simulink model "DvrSimKeybd_cs"  (R2016a)
settings: Solver=ode5  SolverMode=SingleTasking  StartTime=0.0  StopTime=10  FixedStep=1/1000  RelTol=1e-3
PreLoadFcn:
  | mbxruntime.callbacks.PreLoadFcn(bdroot);
PostLoadFcn:
  | mbxruntime.callbacks.PostLoadFcn(bdroot);
InitFcn:
  | mbxruntime.callbacks.InitFcn(bdroot);
StartFcn:
  | mbxruntime.callbacks.StartFcn(bdroot);
StopFcn:
  | mbxruntime.callbacks.StopFcn(bdroot);
model workspace (MAT data in the model file):
  mbox_table : struct (value not decoded)
  model_closed = 0
  sim_status = 0
values from neighbouring files (symbols this model uses):
  CCCDuration = 5    [PreScan_Runscript.m]
  V0 = CCCArray(2*CCCCasei-1)    [PreScan_Runscript.m]
  V1 = CCCArray(2*CCCCasei)    [PreScan_Runscript.m]
  VAccuracyIn = 0.8    [PreScan_Runscript.m]
  VDurationIn = 2    [PreScan_Runscript.m]
  VPIDIn = CCCArray(2*CCCCasei-1)    [PreScan_Runscript.m]
  VToleranceIn = 1    [PreScan_Runscript.m]
undefined symbols (not defined in the file or in its folder): ADASID, BMotor1, BMotor2, BrkDelayTime, DControlB, Delay1, Delay2, DiscIntNeverNeededParam, IControlB, JMotor1, JMotor2, PControlB, PreScanCarSimLoadFcn, ratioGearF, ratioGearR, TorqDelayTime, Tstep
undefined symbols (not defined in the file): WheelL0, WheelL1, WheelR0, WheelR1
libraries: simulink x13, simulink_extras x10, MyLib x3, PreScanSimulinkLibrary x3, Solver_SF x2, pil_lib x1
(part 8 of 9)

== system DvrSimKeybd_cs/Roewe_550_S_Sedan_1/CarSim I//O/PreScanLaneMarker/Subsystem/Sensor Data4 ==
  Sensor Data : Inport
  Bus Selector : BusSelector  OutputSignals=ScanAtSensor.LeftLaneIntersection2.WorldCoordinateY,ScanAtDistance1.LeftLaneIntersection2.WorldCoordinateY,ScanAtDistance2.LeftLaneIntersection2.WorldCoordinateY,ScanAtDistance3.LeftLaneIntersection2.WorldCoordinateY
  Bus Selector1 : BusSelector  OutputSignals=ScanAtSensor.LeftLaneIntersection1.WorldCoordinateY,ScanAtDistance1.LeftLaneIntersection1.WorldCoordinateY,ScanAtDistance2.LeftLaneIntersection1.WorldCoordinateY,ScanAtDistance3.LeftLaneIntersection1.WorldCoordinateY
  Bus Selector2 : BusSelector  OutputSignals=ScanAtSensor.RightLaneIntersection1.WorldCoordinateY,ScanAtDistance1.RightLaneIntersection1.WorldCoordinateY,ScanAtDistance2.RightLaneIntersection1.WorldCoordinateY,ScanAtDistance3.RightLaneIntersection1.WorldCoordinateY
  Bus Selector3 : BusSelector  OutputSignals=ScanAtSensor.RightLaneIntersection2.WorldCoordinateX,ScanAtDistance1.RightLaneIntersection2.WorldCoordinateX,ScanAtDistance2.RightLaneIntersection2.WorldCoordinateX,ScanAtDistance3.RightLaneIntersection2.WorldCoordinateX
  Bus Selector5 : BusSelector  OutputSignals=ScanAtSensor.LeftLaneIntersection2.WorldCoordinateX,ScanAtDistance1.LeftLaneIntersection2.WorldCoordinateX,ScanAtDistance2.LeftLaneIntersection2.WorldCoordinateX,ScanAtDistance3.LeftLaneIntersection2.WorldCoordinateX
  Bus Selector6 : BusSelector  OutputSignals=ScanAtSensor.LeftLaneIntersection1.WorldCoordinateX,ScanAtDistance1.LeftLaneIntersection1.WorldCoordinateX,ScanAtDistance2.LeftLaneIntersection1.WorldCoordinateX,ScanAtDistance3.LeftLaneIntersection1.WorldCoordinateX
  Bus Selector7 : BusSelector  OutputSignals=ScanAtSensor.RightLaneIntersection1.WorldCoordinateX,ScanAtDistance1.RightLaneIntersection1.WorldCoordinateX,ScanAtDistance2.RightLaneIntersection1.WorldCoordinateX,ScanAtDistance3.RightLaneIntersection1.WorldCoordinateX
  Bus Selector8 : BusSelector  OutputSignals=ScanAtSensor.RightLaneIntersection2.WorldCoordinateY,ScanAtDistance1.RightLaneIntersection2.WorldCoordinateY,ScanAtDistance2.RightLaneIntersection2.WorldCoordinateY,ScanAtDistance3.RightLaneIntersection2.WorldCoordinateY
  Mux{,1..7} (8 alike) : Mux
  Lane3_X_Part4 : Outport
  Lane1_X_Part4 : Outport  Port=2
  Lane2_X_Part4 : Outport  Port=3
  Lane4_X_Part4 : Outport  Port=4
  Lane3_Y_Part4 : Outport  Port=5
  Lane1_Y_Part4 : Outport  Port=6
  Lane2_Y_Part4 : Outport  Port=7
  Lane4_Y_Part4 : Outport  Port=8
  wires:
  Sensor Data/1 -> Bus Selector8/1, Bus Selector2/1, Bus Selector1/1, Bus Selector/1, Bus Selector3/1, Bus Selector5/1, Bus Selector6/1, Bus Selector7/1
  Bus Selector5/2 -> Mux/2  "<WorldCoordinateX>"
  Bus Selector5/4 -> Mux/4  "<WorldCoordinateX>"
  Bus Selector5/1 -> Mux/1  "<WorldCoordinateX>"
  Bus Selector5/3 -> Mux/3  "<WorldCoordinateX>"
  Bus Selector/3 -> Mux4/3  "<WorldCoordinateY>"
  Bus Selector/4 -> Mux4/4  "<WorldCoordinateY>"
  Bus Selector/1 -> Mux4/1  "<WorldCoordinateY>"
  Bus Selector/2 -> Mux4/2  "<WorldCoordinateY>"
  Mux/1 -> Lane3_X_Part4/1
  Mux4/1 -> Lane3_Y_Part4/1
  Bus Selector6/4 -> Mux5/4  "<WorldCoordinateX>"
  Bus Selector6/3 -> Mux5/3  "<WorldCoordinateX>"
  Bus Selector6/2 -> Mux5/2  "<WorldCoordinateX>"
  Bus Selector6/1 -> Mux5/1  "<WorldCoordinateX>"
  Bus Selector1/3 -> Mux1/3  "<WorldCoordinateY>"
  Bus Selector1/2 -> Mux1/2  "<WorldCoordinateY>"
  Bus Selector1/4 -> Mux1/4  "<WorldCoordinateY>"
  Bus Selector1/1 -> Mux1/1  "<WorldCoordinateY>"
  Mux1/1 -> Lane1_Y_Part4/1
  Mux5/1 -> Lane1_X_Part4/1
  Bus Selector7/2 -> Mux2/2  "<WorldCoordinateX>"
  Bus Selector7/3 -> Mux2/3  "<WorldCoordinateX>"
  Bus Selector7/1 -> Mux2/1  "<WorldCoordinateX>"
  Bus Selector7/4 -> Mux2/4  "<WorldCoordinateX>"
  Bus Selector2/2 -> Mux3/2  "<WorldCoordinateY>"
  Bus Selector2/1 -> Mux3/1  "<WorldCoordinateY>"
  Bus Selector2/3 -> Mux3/3  "<WorldCoordinateY>"
  Bus Selector2/4 -> Mux3/4  "<WorldCoordinateY>"
  Bus Selector3/2 -> Mux6/2  "<WorldCoordinateX>"
  Bus Selector3/1 -> Mux6/1  "<WorldCoordinateX>"
  Bus Selector3/3 -> Mux6/3  "<WorldCoordinateX>"
  Bus Selector3/4 -> Mux6/4  "<WorldCoordinateX>"
  Bus Selector8/1 -> Mux7/1  "<WorldCoordinateY>"
  Bus Selector8/2 -> Mux7/2  "<WorldCoordinateY>"
  Bus Selector8/3 -> Mux7/3  "<WorldCoordinateY>"
  Bus Selector8/4 -> Mux7/4  "<WorldCoordinateY>"
  Mux3/1 -> Lane2_Y_Part4/1
  Mux7/1 -> Lane4_Y_Part4/1
  Mux2/1 -> Lane2_X_Part4/1
  Mux6/1 -> Lane4_X_Part4/1

== system DvrSimKeybd_cs/Roewe_550_S_Sedan_1/CarSim_Vehicle/CarSim2PreScan_BUS/Steering/AvoidDivisionByZero ==
  In1 : Inport
  Compare To Zero : simulink/Logic and Bit Operations/Compare To Zero  relop===  OutDataTypeStr=uint8
  Constant : Constant  Value=eps
  Product : Product  RndMeth=Zero
  Sum : Sum
  Out1 : Outport
  wires:
  In1/1 -> Compare To Zero/1, Sum/1
  Sum/1 -> Out1/1
  Product/1 -> Sum/2
  Constant/1 -> Product/2
  Compare To Zero/1 -> Product/1

== system DvrSimKeybd_cs/Roewe_550_S_Sedan_1/CarSim_Vehicle/CarSim2PreScan_BUS/Wheel/Convert CarSim to PreScan Wheel Position ==
  SprungMass_Pos_Global[x;y;z][m] : Inport
  SprungMass_Angle_Global[x;y;z][deg] : Inport  Port=2
  CarSim_Pos_FL_Wheel[x;y;z][m] : Inport  Port=3
  CarSim_Pos_FR_Wheel[x;y;z][m] : Inport  Port=4
  CarSim_Pos_RL_Wheel[x;y;z][m] : Inport  Port=5
  CarSim_Pos_RR_Wheel[x;y;z][m] : Inport  Port=6
  Bus Creator1 : BusCreator  Inputs=4
  Demux1 : Demux  Outputs=[3 3 3 3]
  Mux1 : Mux
  Transformation_WheelGlobal2WheelLocal : Subsystem
  PreScanWheel_Pos : Outport
  wires:
  SprungMass_Angle_Global[x;y;z][deg]/1 -> Transformation_WheelGlobal2WheelLocal/2(SprungMass_Angle_Global[x;y;z][deg])
  SprungMass_Pos_Global[x;y;z][m]/1 -> Transformation_WheelGlobal2WheelLocal/1(SprungMass_Pos_Global[x;y;z][m])
  CarSim_Pos_RR_Wheel[x;y;z][m]/1 -> Mux1/4
  CarSim_Pos_RL_Wheel[x;y;z][m]/1 -> Mux1/3
  CarSim_Pos_FR_Wheel[x;y;z][m]/1 -> Mux1/2
  CarSim_Pos_FL_Wheel[x;y;z][m]/1 -> Mux1/1
  Mux1/1 -> Transformation_WheelGlobal2WheelLocal/3(Wheels_Pos_Global[x;y;z][m])
  Bus Creator1/1 -> PreScanWheel_Pos/1  "Linear"
  Demux1/4 -> Bus Creator1/4  "Pos_RR_Wheel_CoorSys_V[x;y;z][m]"
  Demux1/3 -> Bus Creator1/3  "Pos_RL_Wheel_CoorSys_V[x;y;z][m]"
  Demux1/2 -> Bus Creator1/2  "Pos_FR_Wheel_CoorSys_V[x;y;z][m]"
  Demux1/1 -> Bus Creator1/1  "Pos_FL_Wheel_CoorSys_V[x;y;z][m]"
  Transformation_WheelGlobal2WheelLocal/1(Pos_[FL;FR;RL;RR]_Wheel_CoorSys_V[x;y;z][m]) -> Demux1/1

== system DvrSimKeybd_cs/Roewe_550_S_Sedan_1/CarSim_Vehicle/CarSim2PreScan_BUS/Wheel/Convert CarSim to PreScan Wheel Rotation ==
  CarSim_Angle_FL_Wheel_CoorSys_V[deg;rev;deg] : Inport
  CarSim_Angle_FR_Wheel_CoorSys_V[deg;rev;deg] : Inport  Port=2
  CarSim_Angle_RL_Wheel_CoorSys_V[deg;rev;deg] : Inport  Port=3
  CarSim_Angle_RR_Wheel_CoorSys_V[deg;rev;deg] : Inport  Port=4
  Angle_Vehicle[x;y;z][deg] : Inport  Port=5
  Bus Creator{,1,3..4} (4 alike) : BusCreator  Inputs=3
  Bus Creator2 : BusCreator  Inputs=4
  Demux{,1..4} (5 alike) : Demux  Outputs=3
  Rev2D{,1..3} (4 alike) : Gain  Gain=360
  Sum{1..4} (4 alike) : Sum  Inputs=+-
  Terminator : Terminator
  Terminator1 : Terminator
  PreScanWheel_Rot : Outport
  wires:
  [VehicleRoll_deg] -> Sum3/2
  Sum3/1 -> Bus Creator4/1  "Angle_Camber_RR_Wheel_CoorSys_V[deg]"
  [VehicleRoll_deg] -> Sum2/2
  Sum1/1 -> Bus Creator1/1  "Angle_Camber_FR_Wheel_CoorSys_V[deg]"
  [VehicleRoll_deg] -> Sum1/2
  [VehicleRoll_deg] -> Sum4/2
  Demux4/3 -> Terminator1/1
  Demux4/2 -> Terminator/1
  Demux4/1 -> [VehicleRoll_deg]
  Angle_Vehicle[x;y;z][deg]/1 -> Demux4/1
  Rev2D3/1 -> Bus Creator4/2  "Angle_Rot_RR_Wheel[deg]"
  Rev2D2/1 -> Bus Creator3/2  "Angle_Rot_RL_Wheel[deg]"
  Rev2D1/1 -> Bus Creator1/2  "Angle_Rot_FR_Wheel[deg]"
  Rev2D/1 -> Bus Creator/2  "Angle_Rot_FL_Wheel[deg]"
  CarSim_Angle_RR_Wheel_CoorSys_V[deg;rev;deg]/1 -> Demux3/1
  CarSim_Angle_RL_Wheel_CoorSys_V[deg;rev;deg]/1 -> Demux2/1
  CarSim_Angle_FR_Wheel_CoorSys_V[deg;rev;deg]/1 -> Demux1/1
  Demux/1 -> Sum4/1  "CarSImAngle_Camber_FL_Wheel_CoorSys_V[deg]"
  Bus Creator2/1 -> PreScanWheel_Rot/1  "Angualr"
  Bus Creator4/1 -> Bus Creator2/4  "Rot_RR_Wheel_CoorSys_V[x;y;z][deg]"
  Bus Creator3/1 -> Bus Creator2/3  "Rot_RL_Wheel_CoorSys_V[x;y;z][deg]"
  Bus Creator1/1 -> Bus Creator2/2  "Rot_FR_Wheel_CoorSys_V[x;y;z][deg]"
  Bus Creator/1 -> Bus Creator2/1  "Rot_FL_Wheel_CoorSys_V[x;y;z][deg]"
  Demux3/3 -> Bus Creator4/3  "Angle_Toe_RR_Wheel_CoorSys_V[deg]"
  Demux1/3 -> Bus Creator1/3  "Angle_Toe_FR_Wheel_CoorSys_V[deg]"
  Demux2/3 -> Bus Creator3/3  "Angle_Toe_RL_Wheel_CoorSys_V[deg]"
  Sum2/1 -> Bus Creator3/1  "Angle_Camber_RL_Wheel_CoorSys_V[deg]"
  Sum4/1 -> Bus Creator/1  "Angle_Camber_FL_Wheel_CoorSys_V[deg]"
  Demux3/2 -> Rev2D3/1  "Angle_Rot_RR_Wheel[rev]"
  Demux3/1 -> Sum3/1  "Angle_Camber_RR_Wheel_CoorSys_V[deg]"
  Demux2/2 -> Rev2D2/1  "Angle_Rot_RL_Wheel[rev]"
  Demux2/1 -> Sum2/1  "Angle_Camber_RL_Wheel_CoorSys_V[deg]"
  Demux1/2 -> Rev2D1/1  "Angle_Rot_FR_Wheel[rev]"
  Demux1/1 -> Sum1/1  "Angle_Camber_FR_Wheel_CoorSys_V[deg]"
  Demux/3 -> Bus Creator/3  "Angle_Toe_FL_Wheel_CoorSys_V[deg]"
  Demux/2 -> Rev2D/1  "Angle_Rot_FL_Wheel[rev]"
  CarSim_Angle_FL_Wheel_CoorSys_V[deg;rev;deg]/1 -> Demux/1

== system DvrSimKeybd_cs/Roewe_550_S_Sedan_1/CarSim_Vehicle/TyreContact To Road Information/Contact To Road Information/AvoidDivisionByZero ==
  In1 : Inport
  Compare To Zero : simulink/Logic and Bit Operations/Compare To Zero  relop===  OutDataTypeStr=uint8
  Constant : Constant  Value=eps
  Product : Product  RndMeth=Zero
  Sum : Sum
  Out1 : Outport
  wires:
  In1/1 -> Compare To Zero/1, Sum/1
  Sum/1 -> Out1/1
  Product/1 -> Sum/2
  Constant/1 -> Product/2
  Compare To Zero/1 -> Product/1

== system DvrSimKeybd_cs/Roewe_550_S_Sedan_1/CarSim_Vehicle/TyreContact To Road Information/Contact To Road Information/Transformation_PreScan2CarSim ==
  UnitVec_z_CP_CoorSys_PreScan[FL;FR;RL;RR][x;y;z] : Inport
  angles_BODYwrtGLOB_[deg] : Inport  Port=2
  Bus Creator : BusCreator  Inputs=4
  D2R : Gain  Gain=pi/180
  Fcn1 : Fcn  Expr=cos(u(1))*sin(u(2))*sin(u(3))-sin(u(1))*cos(u(3))
  Fcn18 : Fcn  Expr=cos(u(1))*cos(u(2))
  Fcn2 : Fcn  Expr=cos(u(1))*sin(u(2))*cos(u(3))+sin(u(1))*sin(u(3))
  Fcn3 : Fcn  Expr=sin(u(1))*cos(u(2))
  Fcn4 : Fcn  Expr=sin(u(1))*sin(u(2))*sin(u(3))+cos(u(1))*cos(u(3))
  Fcn5 : Fcn  Expr=sin(u(1))*sin(u(2))*cos(u(3))-cos(u(1))*sin(u(3))
  Fcn6 : Fcn  Expr=-sin(u(2))
  Fcn7 : Fcn  Expr=cos(u(2))*sin(u(3))
  Fcn8 : Fcn  Expr=cos(u(2))*cos(u(3))
  Mux2 : Mux  Inputs=9
  Selector : Selector  InputPortWidth=9  IndexOptions=Index vector (dialog)  Indices=[1 2 3]  OutputSizes=1
  Selector1 : Selector  InputPortWidth=9  IndexOptions=Index vector (dialog)  Indices=[4 5 6]  OutputSizes=1
  Selector2 : Selector  InputPortWidth=9  IndexOptions=Index vector (dialog)  Indices=[7 8 9]  OutputSizes=1
  Subsystem : Subsystem
  rot_xyz 2 rot_zyx : Selector  InputPortWidth=3  IndexOptions=Index vector (dialog)  Indices=[3 2 1]  OutputSizes=1
  UnitVec_z_CP_CoorSys _CarSim[FL;FR;RL;RR][x;y;z] : Outport
  wires:
  Fcn18/1 -> Mux2/1
  Fcn3/1 -> Mux2/2
  Fcn6/1 -> Mux2/3
  Fcn1/1 -> Mux2/4
  Fcn4/1 -> Mux2/5
  Fcn7/1 -> Mux2/6
  Fcn2/1 -> Mux2/7
  Fcn5/1 -> Mux2/8
  Fcn8/1 -> Mux2/9
  Mux2/1 -> Selector/1, Selector1/1, Selector2/1  "Inverse RotationMatrix"
  rot_xyz 2 rot_zyx/1 -> Fcn18/1, Fcn3/1, Fcn6/1, Fcn1/1, Fcn4/1, Fcn8/1, Fcn5/1, Fcn2/1, Fcn7/1
  D2R/1 -> rot_xyz 2 rot_zyx/1
  Subsystem/4(UnitVec_z_CP_CoorSys_CarSim[RR][x;y;z]) -> Bus Creator/4
  Subsystem/3(UnitVec_z_CP_CoorSys_CarSim[RL][x;y;z]) -> Bus Creator/3
  Subsystem/2(UnitVec_z_CP_CoorSys_CarSim[FR][x;y;z]) -> Bus Creator/2
  Subsystem/1(UnitVec_z_CP_CoorSys_CarSim[FL][x;y;z]) -> Bus Creator/1
  UnitVec_z_CP_CoorSys_PreScan[FL;FR;RL;RR][x;y;z]/1 -> Subsystem/1(UnitVec_z_CP_CoorSys_PreScan[FL;FR;RL;RR][x;y;z])
  angles_BODYwrtGLOB_[deg]/1 -> D2R/1
  Bus Creator/1 -> UnitVec_z_CP_CoorSys _CarSim[FL;FR;RL;RR][x;y;z]/1
  Selector2/1 -> Subsystem/4(ThirdRow)
  Selector1/1 -> Subsystem/3(SecondRow)
  Selector/1 -> Subsystem/2(FirstRow)

== system DvrSimKeybd_cs/Roewe_550_S_Sedan_1/PreScan_RayCast_Contact_Sensor/Vehicle Local to World/state2FullState/Transformation_BODY2GLOBAL1 ==
  POSvector_BODY_[m] : Inport
  angles_BODYwrtGLOB_[rad] : Inport  Port=2
  Dot Product : DotProduct  InputSameDT=on  OutDataTypeStr=Inherit: Inherit via internal rule
  Dot Product1 : DotProduct  InputSameDT=on  OutDataTypeStr=Inherit: Inherit via internal rule
  Dot Product2 : DotProduct  InputSameDT=on  OutDataTypeStr=Inherit: Inherit via internal rule
  Fcn10 : Fcn  Expr=cos(u(1))*sin(u(2))*sin(u(3))-sin(u(1))*cos(u(3))
  Fcn11 : Fcn  Expr=cos(u(1))*sin(u(2))*cos(u(3))+sin(u(1))*sin(u(3))
  Fcn12 : Fcn  Expr=sin(u(1))*cos(u(2))
  Fcn13 : Fcn  Expr=sin(u(1))*sin(u(2))*sin(u(3))+cos(u(1))*cos(u(3))
  Fcn14 : Fcn  Expr=sin(u(1))*sin(u(2))*cos(u(3))-cos(u(1))*sin(u(3))
  Fcn15 : Fcn  Expr=-sin(u(2))
  Fcn16 : Fcn  Expr=cos(u(2))*sin(u(3))
  Fcn17 : Fcn  Expr=cos(u(2))*cos(u(3))
  Fcn9 : Fcn  Expr=cos(u(1))*cos(u(2))
  Mux1 : Mux  Inputs=9
  Mux3 : Mux  Inputs=3
  Selector : Selector  InputPortWidth=9  IndexOptions=Index vector (dialog)  Indices=[1 2 3]  OutputSizes=1
  Selector1 : Selector  InputPortWidth=9  IndexOptions=Index vector (dialog)  Indices=[4 5 6]  OutputSizes=1
  Selector2 : Selector  InputPortWidth=9  IndexOptions=Index vector (dialog)  Indices=[7 8 9]  OutputSizes=1
  rot_xyz 2 rot_zyx : Selector  InputPortWidth=3  IndexOptions=Index vector (dialog)  Indices=[3 2 1]  OutputSizes=1
  POSvector_GLOBAL_[m] : Outport
  wires:
  angles_BODYwrtGLOB_[rad]/1 -> rot_xyz 2 rot_zyx/1
  Mux3/1 -> POSvector_GLOBAL_[m]/1
  rot_xyz 2 rot_zyx/1 -> Fcn17/1, Fcn16/1, Fcn15/1, Fcn14/1, Fcn13/1, Fcn12/1, Fcn11/1, Fcn10/1, Fcn9/1
  Dot Product1/1 -> Mux3/2
  Dot Product2/1 -> Mux3/3
  Selector2/1 -> Dot Product2/2
  Selector1/1 -> Dot Product1/2
  Dot Product/1 -> Mux3/1
  POSvector_BODY_[m]/1 -> Dot Product/1, Dot Product1/1, Dot Product2/1
  Selector/1 -> Dot Product/2
  Mux1/1 -> Selector2/1, Selector1/1, Selector/1  "RotationMatrix"
  Fcn17/1 -> Mux1/9
  Fcn16/1 -> Mux1/8
  Fcn15/1 -> Mux1/7
  Fcn14/1 -> Mux1/6
  Fcn13/1 -> Mux1/5
  Fcn12/1 -> Mux1/4
  Fcn11/1 -> Mux1/3
  Fcn10/1 -> Mux1/2
  Fcn9/1 -> Mux1/1

== system DvrSimKeybd_cs/Roewe_550_S_Sedan_1/PreScan_RayCast_Contact_Sensor/Vehicle Local to World/state2FullState/limit roll ==
  RPY : Inport
  Demux : Demux  Outputs=3
  Mux1 : Mux  Inputs=3
  Substitute 90 & 270 deg (and its plurals) : Subsystem
  RPYcor : Outport
  wires:
  Demux/1 -> Substitute 90 & 270 deg (and its plurals)/1(Angle [rad])
  Demux/2 -> Mux1/2
  Demux/3 -> Mux1/3
  RPY/1 -> Demux/1
  Mux1/1 -> RPYcor/1
  Substitute 90 & 270 deg (and its plurals)/1(Subst Angle [rad]) -> Mux1/1

== system DvrSimKeybd_cs/Roewe_550_S_Sedan_1/PreScan_RayCast_Contact_Sensor/Wheels Local to World/conv_RotWheelFL/RotMat2AxisAngle ==
  RotMat_Visu : Inport
  Data Type Conversion : DataTypeConversion
  Divide : Product  Inputs=*/
  Gain : Gain  Gain=2
  Mux : Mux  Inputs=3
  Mux1 : Mux  Inputs=2
  Saturation1 : Saturate  UpperLimit=3-0.001  LowerLimit=-1+0.001
  Trigonometric Function : Trigonometry
  U1 : Fcn  Expr=u[6]-u[8]
  U2 : Fcn  Expr=u[7]-u[3]
  U3 : Fcn  Expr=u[2]-u[4]
  U_Phi : Fcn  Expr=u[1]+u[5]+u[9]
  U_Phi1 : Fcn  Expr=acos((u(1)-1)/2)
  U_Phi2 : Fcn  Expr=acos((u(1)-1)/2)
  Angles_Visu : Outport
  wires:
  Data Type Conversion/1 -> Mux1/2
  RotMat_Visu/1 -> U1/1, U2/1, U3/1, U_Phi/1
  Trigonometric Function/1 -> Gain/1
  U1/1 -> Mux/1
  U2/1 -> Mux/2
  U3/1 -> Mux/3
  Mux/1 -> Divide/1
  Gain/1 -> Divide/2
  Mux1/1 -> Angles_Visu/1
  Divide/1 -> Mux1/1
  U_Phi/1 -> U_Phi1/1, Saturation1/1
  U_Phi1/1 -> Data Type Conversion/1
  Saturation1/1 -> U_Phi2/1
  U_Phi2/1 -> Trigonometric Function/1

== system DvrSimKeybd_cs/Roewe_550_S_Sedan_1/PreScan_RayCast_Contact_Sensor/Wheels Local to World/conv_RotWheelFR/RotMat2AxisAngle ==
  RotMat_Visu : Inport
  Data Type Conversion : DataTypeConversion
  Divide : Product  Inputs=*/
  Gain : Gain  Gain=2
  Mux : Mux  Inputs=3
  Mux1 : Mux  Inputs=2
  Saturation1 : Saturate  UpperLimit=3-0.001  LowerLimit=-1+0.001
  Trigonometric Function : Trigonometry
  U1 : Fcn  Expr=u[6]-u[8]
  U2 : Fcn  Expr=u[7]-u[3]
  U3 : Fcn  Expr=u[2]-u[4]
  U_Phi : Fcn  Expr=u[1]+u[5]+u[9]
  U_Phi1 : Fcn  Expr=acos((u(1)-1)/2)
  U_Phi2 : Fcn  Expr=acos((u(1)-1)/2)
  Angles_Visu : Outport
  wires:
  U_Phi2/1 -> Trigonometric Function/1
  Saturation1/1 -> U_Phi2/1
  U_Phi1/1 -> Data Type Conversion/1
  U_Phi/1 -> Saturation1/1, U_Phi1/1
  Divide/1 -> Mux1/1
  Mux1/1 -> Angles_Visu/1
  Gain/1 -> Divide/2
  Mux/1 -> Divide/1
  U3/1 -> Mux/3
  U2/1 -> Mux/2
  U1/1 -> Mux/1
  Trigonometric Function/1 -> Gain/1
  RotMat_Visu/1 -> U_Phi/1, U3/1, U2/1, U1/1
  Data Type Conversion/1 -> Mux1/2

== system DvrSimKeybd_cs/Roewe_550_S_Sedan_1/PreScan_RayCast_Contact_Sensor/Wheels Local to World/conv_RotWheelRL/RotMat2AxisAngle ==
  RotMat_Visu : Inport
  Data Type Conversion : DataTypeConversion
  Divide : Product  Inputs=*/
  Gain : Gain  Gain=2
  Mux : Mux  Inputs=3
  Mux1 : Mux  Inputs=2
  Saturation1 : Saturate  UpperLimit=3-0.001  LowerLimit=-1+0.001
  Trigonometric Function : Trigonometry
  U1 : Fcn  Expr=u[6]-u[8]
  U2 : Fcn  Expr=u[7]-u[3]
  U3 : Fcn  Expr=u[2]-u[4]
  U_Phi : Fcn  Expr=u[1]+u[5]+u[9]
  U_Phi1 : Fcn  Expr=acos((u(1)-1)/2)
  U_Phi2 : Fcn  Expr=acos((u(1)-1)/2)
  Angles_Visu : Outport
  wires:
  U_Phi2/1 -> Trigonometric Function/1
  Saturation1/1 -> U_Phi2/1
  U_Phi1/1 -> Data Type Conversion/1
  U_Phi/1 -> Saturation1/1, U_Phi1/1
  Divide/1 -> Mux1/1
  Mux1/1 -> Angles_Visu/1
  Gain/1 -> Divide/2
  Mux/1 -> Divide/1
  U3/1 -> Mux/3
  U2/1 -> Mux/2
  U1/1 -> Mux/1
  Trigonometric Function/1 -> Gain/1
  RotMat_Visu/1 -> U_Phi/1, U3/1, U2/1, U1/1
  Data Type Conversion/1 -> Mux1/2

== system DvrSimKeybd_cs/Roewe_550_S_Sedan_1/PreScan_RayCast_Contact_Sensor/Wheels Local to World/conv_RotWheelRR/RotMat2AxisAngle ==
  RotMat_Visu : Inport
  Data Type Conversion : DataTypeConversion
  Divide : Product  Inputs=*/
  Gain : Gain  Gain=2
  Mux : Mux  Inputs=3
  Mux1 : Mux  Inputs=2
  Saturation1 : Saturate  UpperLimit=3-0.001  LowerLimit=-1+0.001
  Trigonometric Function : Trigonometry
  U1 : Fcn  Expr=u[6]-u[8]
  U2 : Fcn  Expr=u[7]-u[3]
  U3 : Fcn  Expr=u[2]-u[4]
  U_Phi : Fcn  Expr=u[1]+u[5]+u[9]
  U_Phi1 : Fcn  Expr=acos((u(1)-1)/2)
  U_Phi2 : Fcn  Expr=acos((u(1)-1)/2)
  Angles_Visu : Outport
  wires:
  U_Phi2/1 -> Trigonometric Function/1
  Saturation1/1 -> U_Phi2/1
  U_Phi1/1 -> Data Type Conversion/1
  U_Phi/1 -> Saturation1/1, U_Phi1/1
  Divide/1 -> Mux1/1
  Mux1/1 -> Angles_Visu/1
  Gain/1 -> Divide/2
  Mux/1 -> Divide/1
  U3/1 -> Mux/3
  U2/1 -> Mux/2
  U1/1 -> Mux/1
  Trigonometric Function/1 -> Gain/1
  RotMat_Visu/1 -> U_Phi/1, U3/1, U2/1, U1/1
  Data Type Conversion/1 -> Mux1/2

== system DvrSimKeybd_cs/Roewe_550_S_Sedan_1/PreScan_RayCast_Contact_Sensor/Wheels Local to World/conv_TransWheelFL/pos_ini_Visu ==
  Constant : Constant  Value=x_ini_VRML
  Constant1 : Constant  Value=y_ini_VRML
  Constant2 : Constant  Value=z_ini_VRML
  Mux1 : Mux  Inputs=3
  pos_ini_Visu : Outport
  wires:
  Constant/1 -> Mux1/1
  Mux1/1 -> pos_ini_Visu/1
  Constant1/1 -> Mux1/2
  Constant2/1 -> Mux1/3

== system DvrSimKeybd_cs/Roewe_550_S_Sedan_1/PreScan_RayCast_Contact_Sensor/Wheels Local to World/conv_TransWheelFL/transISO2Visu ==
  transISO : Inport
  Demux : Demux  Outputs=3
  trans_x_Visu : Outport
  trans_y_Visu : Outport  Port=2
  trans_z_Visu : Outport  Port=3
  wires:
  Demux/2 -> trans_y_Visu/1  "rot_y"
  Demux/1 -> trans_x_Visu/1
  transISO/1 -> Demux/1
  Demux/3 -> trans_z_Visu/1

== system DvrSimKeybd_cs/Roewe_550_S_Sedan_1/PreScan_RayCast_Contact_Sensor/Wheels Local to World/conv_TransWheelFR/pos_ini_Visu ==
  Constant : Constant  Value=x_ini_VRML
  Constant1 : Constant  Value=y_ini_VRML
  Constant2 : Constant  Value=z_ini_VRML
  Mux1 : Mux  Inputs=3
  pos_ini_Visu : Outport
  wires:
  Constant2/1 -> Mux1/3
  Constant1/1 -> Mux1/2
  Mux1/1 -> pos_ini_Visu/1
  Constant/1 -> Mux1/1

== system DvrSimKeybd_cs/Roewe_550_S_Sedan_1/PreScan_RayCast_Contact_Sensor/Wheels Local to World/conv_TransWheelFR/transISO2Visu ==
  transISO : Inport
  Demux : Demux  Outputs=3
  trans_x_Visu : Outport
  trans_y_Visu : Outport  Port=2
  trans_z_Visu : Outport  Port=3
  wires:
  Demux/2 -> trans_y_Visu/1  "rot_y"
  Demux/1 -> trans_x_Visu/1
  transISO/1 -> Demux/1
  Demux/3 -> trans_z_Visu/1

== system DvrSimKeybd_cs/Roewe_550_S_Sedan_1/PreScan_RayCast_Contact_Sensor/Wheels Local to World/conv_TransWheelRL/pos_ini_Visu ==
  Constant : Constant  Value=x_ini_VRML
  Constant1 : Constant  Value=y_ini_VRML
  Constant2 : Constant  Value=z_ini_VRML
  Mux1 : Mux  Inputs=3
  pos_ini_Visu : Outport
  wires:
  Constant2/1 -> Mux1/3
  Constant1/1 -> Mux1/2
  Mux1/1 -> pos_ini_Visu/1
  Constant/1 -> Mux1/1

== system DvrSimKeybd_cs/Roewe_550_S_Sedan_1/PreScan_RayCast_Contact_Sensor/Wheels Local to World/conv_TransWheelRL/transISO2Visu ==
  transISO : Inport
  Demux : Demux  Outputs=3
  trans_x_Visu : Outport
  trans_y_Visu : Outport  Port=2
  trans_z_Visu : Outport  Port=3
  wires:
  Demux/2 -> trans_y_Visu/1  "rot_y"
  Demux/1 -> trans_x_Visu/1
  transISO/1 -> Demux/1
  Demux/3 -> trans_z_Visu/1

== system DvrSimKeybd_cs/Roewe_550_S_Sedan_1/PreScan_RayCast_Contact_Sensor/Wheels Local to World/conv_TransWheelRR/pos_ini_Visu ==
  Constant : Constant  Value=x_ini_VRML
  Constant1 : Constant  Value=y_ini_VRML
  Constant2 : Constant  Value=z_ini_VRML
  Mux1 : Mux  Inputs=3
  pos_ini_Visu : Outport
  wires:
  Constant2/1 -> Mux1/3
  Constant1/1 -> Mux1/2
  Mux1/1 -> pos_ini_Visu/1
  Constant/1 -> Mux1/1

== system DvrSimKeybd_cs/Roewe_550_S_Sedan_1/PreScan_RayCast_Contact_Sensor/Wheels Local to World/conv_TransWheelRR/transISO2Visu ==
  transISO : Inport
  Demux : Demux  Outputs=3
  trans_x_Visu : Outport
  trans_y_Visu : Outport  Port=2
  trans_z_Visu : Outport  Port=3
  wires:
  Demux/2 -> trans_y_Visu/1  "rot_y"
  Demux/1 -> trans_x_Visu/1
  transISO/1 -> Demux/1
  Demux/3 -> trans_z_Visu/1

== system DvrSimKeybd_cs/Roewe_550_S_Sedan_1/PreScan_RayCast_Contact_Sensor1/Vehicle Local to World/state2FullState/Transformation_BODY2GLOBAL1 ==
  POSvector_BODY_[m] : Inport
  angles_BODYwrtGLOB_[rad] : Inport  Port=2
  Dot Product : DotProduct  InputSameDT=on  OutDataTypeStr=Inherit: Inherit via internal rule
  Dot Product1 : DotProduct  InputSameDT=on  OutDataTypeStr=Inherit: Inherit via internal rule
  Dot Product2 : DotProduct  InputSameDT=on  OutDataTypeStr=Inherit: Inherit via internal rule
  Fcn10 : Fcn  Expr=cos(u(1))*sin(u(2))*sin(u(3))-sin(u(1))*cos(u(3))
  Fcn11 : Fcn  Expr=cos(u(1))*sin(u(2))*cos(u(3))+sin(u(1))*sin(u(3))
  Fcn12 : Fcn  Expr=sin(u(1))*cos(u(2))
  Fcn13 : Fcn  Expr=sin(u(1))*sin(u(2))*sin(u(3))+cos(u(1))*cos(u(3))
  Fcn14 : Fcn  Expr=sin(u(1))*sin(u(2))*cos(u(3))-cos(u(1))*sin(u(3))
  Fcn15 : Fcn  Expr=-sin(u(2))
  Fcn16 : Fcn  Expr=cos(u(2))*sin(u(3))
  Fcn17 : Fcn  Expr=cos(u(2))*cos(u(3))
  Fcn9 : Fcn  Expr=cos(u(1))*cos(u(2))
  Mux1 : Mux  Inputs=9
  Mux3 : Mux  Inputs=3
  Selector : Selector  InputPortWidth=9  IndexOptions=Index vector (dialog)  Indices=[1 2 3]  OutputSizes=1
  Selector1 : Selector  InputPortWidth=9  IndexOptions=Index vector (dialog)  Indices=[4 5 6]  OutputSizes=1
  Selector2 : Selector  InputPortWidth=9  IndexOptions=Index vector (dialog)  Indices=[7 8 9]  OutputSizes=1
  rot_xyz 2 rot_zyx : Selector  InputPortWidth=3  IndexOptions=Index vector (dialog)  Indices=[3 2 1]  OutputSizes=1
  POSvector_GLOBAL_[m] : Outport
  wires:
  angles_BODYwrtGLOB_[rad]/1 -> rot_xyz 2 rot_zyx/1
  Mux3/1 -> POSvector_GLOBAL_[m]/1
  rot_xyz 2 rot_zyx/1 -> Fcn17/1, Fcn16/1, Fcn15/1, Fcn14/1, Fcn13/1, Fcn12/1, Fcn11/1, Fcn10/1, Fcn9/1
  Dot Product1/1 -> Mux3/2
  Dot Product2/1 -> Mux3/3
  Selector2/1 -> Dot Product2/2
  Selector1/1 -> Dot Product1/2
  Dot Product/1 -> Mux3/1
  POSvector_BODY_[m]/1 -> Dot Product/1, Dot Product1/1, Dot Product2/1
  Selector/1 -> Dot Product/2
  Mux1/1 -> Selector2/1, Selector1/1, Selector/1  "RotationMatrix"
  Fcn17/1 -> Mux1/9
  Fcn16/1 -> Mux1/8
  Fcn15/1 -> Mux1/7
  Fcn14/1 -> Mux1/6
  Fcn13/1 -> Mux1/5
  Fcn12/1 -> Mux1/4
  Fcn11/1 -> Mux1/3
  Fcn10/1 -> Mux1/2
  Fcn9/1 -> Mux1/1

== system DvrSimKeybd_cs/Roewe_550_S_Sedan_1/PreScan_RayCast_Contact_Sensor1/Vehicle Local to World/state2FullState/limit roll ==
  RPY : Inport
  Demux : Demux  Outputs=3
  Mux1 : Mux  Inputs=3
  Substitute 90 & 270 deg (and its plurals) : Subsystem
  RPYcor : Outport
  wires:
  Demux/1 -> Substitute 90 & 270 deg (and its plurals)/1(Angle [rad])
  Demux/2 -> Mux1/2
  Demux/3 -> Mux1/3
  RPY/1 -> Demux/1
  Mux1/1 -> RPYcor/1
  Substitute 90 & 270 deg (and its plurals)/1(Subst Angle [rad]) -> Mux1/1

== system DvrSimKeybd_cs/Roewe_550_S_Sedan_1/PreScan_RayCast_Contact_Sensor1/Wheels Local to World/conv_RotWheelFL/RotMat2AxisAngle ==
  RotMat_Visu : Inport
  Data Type Conversion : DataTypeConversion
  Divide : Product  Inputs=*/
  Gain : Gain  Gain=2
  Mux : Mux  Inputs=3
  Mux1 : Mux  Inputs=2
  Saturation1 : Saturate  UpperLimit=3-0.001  LowerLimit=-1+0.001
  Trigonometric Function : Trigonometry
  U1 : Fcn  Expr=u[6]-u[8]
  U2 : Fcn  Expr=u[7]-u[3]
  U3 : Fcn  Expr=u[2]-u[4]
  U_Phi : Fcn  Expr=u[1]+u[5]+u[9]
  U_Phi1 : Fcn  Expr=acos((u(1)-1)/2)
  U_Phi2 : Fcn  Expr=acos((u(1)-1)/2)
  Angles_Visu : Outport
  wires:
  Data Type Conversion/1 -> Mux1/2
  RotMat_Visu/1 -> U1/1, U2/1, U3/1, U_Phi/1
  Trigonometric Function/1 -> Gain/1
  U1/1 -> Mux/1
  U2/1 -> Mux/2
  U3/1 -> Mux/3
  Mux/1 -> Divide/1
  Gain/1 -> Divide/2
  Mux1/1 -> Angles_Visu/1
  Divide/1 -> Mux1/1
  U_Phi/1 -> U_Phi1/1, Saturation1/1
  U_Phi1/1 -> Data Type Conversion/1
  Saturation1/1 -> U_Phi2/1
  U_Phi2/1 -> Trigonometric Function/1

== system DvrSimKeybd_cs/Roewe_550_S_Sedan_1/PreScan_RayCast_Contact_Sensor1/Wheels Local to World/conv_RotWheelFR/RotMat2AxisAngle ==
  RotMat_Visu : Inport
  Data Type Conversion : DataTypeConversion
  Divide : Product  Inputs=*/
  Gain : Gain  Gain=2
  Mux : Mux  Inputs=3
  Mux1 : Mux  Inputs=2
  Saturation1 : Saturate  UpperLimit=3-0.001  LowerLimit=-1+0.001
  Trigonometric Function : Trigonometry
  U1 : Fcn  Expr=u[6]-u[8]
  U2 : Fcn  Expr=u[7]-u[3]
  U3 : Fcn  Expr=u[2]-u[4]
  U_Phi : Fcn  Expr=u[1]+u[5]+u[9]
  U_Phi1 : Fcn  Expr=acos((u(1)-1)/2)
  U_Phi2 : Fcn  Expr=acos((u(1)-1)/2)
  Angles_Visu : Outport
  wires:
  U_Phi2/1 -> Trigonometric Function/1
  Saturation1/1 -> U_Phi2/1
  U_Phi1/1 -> Data Type Conversion/1
  U_Phi/1 -> Saturation1/1, U_Phi1/1
  Divide/1 -> Mux1/1
  Mux1/1 -> Angles_Visu/1
  Gain/1 -> Divide/2
  Mux/1 -> Divide/1
  U3/1 -> Mux/3
  U2/1 -> Mux/2
  U1/1 -> Mux/1
  Trigonometric Function/1 -> Gain/1
  RotMat_Visu/1 -> U_Phi/1, U3/1, U2/1, U1/1
  Data Type Conversion/1 -> Mux1/2

== system DvrSimKeybd_cs/Roewe_550_S_Sedan_1/PreScan_RayCast_Contact_Sensor1/Wheels Local to World/conv_RotWheelRL/RotMat2AxisAngle ==
  RotMat_Visu : Inport
  Data Type Conversion : DataTypeConversion
  Divide : Product  Inputs=*/
  Gain : Gain  Gain=2
  Mux : Mux  Inputs=3
  Mux1 : Mux  Inputs=2
  Saturation1 : Saturate  UpperLimit=3-0.001  LowerLimit=-1+0.001
  Trigonometric Function : Trigonometry
  U1 : Fcn  Expr=u[6]-u[8]
  U2 : Fcn  Expr=u[7]-u[3]
  U3 : Fcn  Expr=u[2]-u[4]
  U_Phi : Fcn  Expr=u[1]+u[5]+u[9]
  U_Phi1 : Fcn  Expr=acos((u(1)-1)/2)
  U_Phi2 : Fcn  Expr=acos((u(1)-1)/2)
  Angles_Visu : Outport
  wires:
  U_Phi2/1 -> Trigonometric Function/1
  Saturation1/1 -> U_Phi2/1
  U_Phi1/1 -> Data Type Conversion/1
  U_Phi/1 -> Saturation1/1, U_Phi1/1
  Divide/1 -> Mux1/1
  Mux1/1 -> Angles_Visu/1
  Gain/1 -> Divide/2
  Mux/1 -> Divide/1
  U3/1 -> Mux/3
  U2/1 -> Mux/2
  U1/1 -> Mux/1
  Trigonometric Function/1 -> Gain/1
  RotMat_Visu/1 -> U_Phi/1, U3/1, U2/1, U1/1
  Data Type Conversion/1 -> Mux1/2

== system DvrSimKeybd_cs/Roewe_550_S_Sedan_1/PreScan_RayCast_Contact_Sensor1/Wheels Local to World/conv_RotWheelRR/RotMat2AxisAngle ==
  RotMat_Visu : Inport
  Data Type Conversion : DataTypeConversion
  Divide : Product  Inputs=*/
  Gain : Gain  Gain=2
  Mux : Mux  Inputs=3
  Mux1 : Mux  Inputs=2
  Saturation1 : Saturate  UpperLimit=3-0.001  LowerLimit=-1+0.001
  Trigonometric Function : Trigonometry
  U1 : Fcn  Expr=u[6]-u[8]
  U2 : Fcn  Expr=u[7]-u[3]
  U3 : Fcn  Expr=u[2]-u[4]
  U_Phi : Fcn  Expr=u[1]+u[5]+u[9]
  U_Phi1 : Fcn  Expr=acos((u(1)-1)/2)
  U_Phi2 : Fcn  Expr=acos((u(1)-1)/2)
  Angles_Visu : Outport
  wires:
  U_Phi2/1 -> Trigonometric Function/1
  Saturation1/1 -> U_Phi2/1
  U_Phi1/1 -> Data Type Conversion/1
  U_Phi/1 -> Saturation1/1, U_Phi1/1
  Divide/1 -> Mux1/1
  Mux1/1 -> Angles_Visu/1
  Gain/1 -> Divide/2
  Mux/1 -> Divide/1
  U3/1 -> Mux/3
  U2/1 -> Mux/2
  U1/1 -> Mux/1
  Trigonometric Function/1 -> Gain/1
  RotMat_Visu/1 -> U_Phi/1, U3/1, U2/1, U1/1
  Data Type Conversion/1 -> Mux1/2

== system DvrSimKeybd_cs/Roewe_550_S_Sedan_1/PreScan_RayCast_Contact_Sensor1/Wheels Local to World/conv_TransWheelFL/pos_ini_Visu ==
  Constant : Constant  Value=x_ini_VRML
  Constant1 : Constant  Value=y_ini_VRML
  Constant2 : Constant  Value=z_ini_VRML
  Mux1 : Mux  Inputs=3
  pos_ini_Visu : Outport
  wires:
  Constant/1 -> Mux1/1
  Mux1/1 -> pos_ini_Visu/1
  Constant1/1 -> Mux1/2
  Constant2/1 -> Mux1/3

== system DvrSimKeybd_cs/Roewe_550_S_Sedan_1/PreScan_RayCast_Contact_Sensor1/Wheels Local to World/conv_TransWheelFL/transISO2Visu ==
  transISO : Inport
  Demux : Demux  Outputs=3
  trans_x_Visu : Outport
  trans_y_Visu : Outport  Port=2
  trans_z_Visu : Outport  Port=3
  wires:
  Demux/2 -> trans_y_Visu/1  "rot_y"
  Demux/1 -> trans_x_Visu/1
  transISO/1 -> Demux/1
  Demux/3 -> trans_z_Visu/1

== system DvrSimKeybd_cs/Roewe_550_S_Sedan_1/PreScan_RayCast_Contact_Sensor1/Wheels Local to World/conv_TransWheelFR/pos_ini_Visu ==
  Constant : Constant  Value=x_ini_VRML
  Constant1 : Constant  Value=y_ini_VRML
  Constant2 : Constant  Value=z_ini_VRML
  Mux1 : Mux  Inputs=3
  pos_ini_Visu : Outport
  wires:
  Constant2/1 -> Mux1/3
  Constant1/1 -> Mux1/2
  Mux1/1 -> pos_ini_Visu/1
  Constant/1 -> Mux1/1

== system DvrSimKeybd_cs/Roewe_550_S_Sedan_1/PreScan_RayCast_Contact_Sensor1/Wheels Local to World/conv_TransWheelFR/transISO2Visu ==
  transISO : Inport
  Demux : Demux  Outputs=3
  trans_x_Visu : Outport
  trans_y_Visu : Outport  Port=2
  trans_z_Visu : Outport  Port=3
  wires:
  Demux/2 -> trans_y_Visu/1  "rot_y"
  Demux/1 -> trans_x_Visu/1
  transISO/1 -> Demux/1
  Demux/3 -> trans_z_Visu/1

== system DvrSimKeybd_cs/Roewe_550_S_Sedan_1/PreScan_RayCast_Contact_Sensor1/Wheels Local to World/conv_TransWheelRL/pos_ini_Visu ==
  Constant : Constant  Value=x_ini_VRML
  Constant1 : Constant  Value=y_ini_VRML
  Constant2 : Constant  Value=z_ini_VRML
  Mux1 : Mux  Inputs=3
  pos_ini_Visu : Outport
  wires:
  Constant2/1 -> Mux1/3
  Constant1/1 -> Mux1/2
  Mux1/1 -> pos_ini_Visu/1
  Constant/1 -> Mux1/1

== system DvrSimKeybd_cs/Roewe_550_S_Sedan_1/PreScan_RayCast_Contact_Sensor1/Wheels Local to World/conv_TransWheelRL/transISO2Visu ==
  transISO : Inport
  Demux : Demux  Outputs=3
  trans_x_Visu : Outport
  trans_y_Visu : Outport  Port=2
  trans_z_Visu : Outport  Port=3
  wires:
  Demux/2 -> trans_y_Visu/1  "rot_y"
  Demux/1 -> trans_x_Visu/1
  transISO/1 -> Demux/1
  Demux/3 -> trans_z_Visu/1

== system DvrSimKeybd_cs/Roewe_550_S_Sedan_1/PreScan_RayCast_Contact_Sensor1/Wheels Local to World/conv_TransWheelRR/pos_ini_Visu ==
  Constant : Constant  Value=x_ini_VRML
  Constant1 : Constant  Value=y_ini_VRML
  Constant2 : Constant  Value=z_ini_VRML
  Mux1 : Mux  Inputs=3
  pos_ini_Visu : Outport
  wires:
  Constant2/1 -> Mux1/3
  Constant1/1 -> Mux1/2
  Mux1/1 -> pos_ini_Visu/1
  Constant/1 -> Mux1/1

== system DvrSimKeybd_cs/Roewe_550_S_Sedan_1/PreScan_RayCast_Contact_Sensor1/Wheels Local to World/conv_TransWheelRR/transISO2Visu ==
  transISO : Inport
  Demux : Demux  Outputs=3
  trans_x_Visu : Outport
  trans_y_Visu : Outport  Port=2
  trans_z_Visu : Outport  Port=3
  wires:
  Demux/2 -> trans_y_Visu/1  "rot_y"
  Demux/1 -> trans_x_Visu/1
  transISO/1 -> Demux/1
  Demux/3 -> trans_z_Visu/1

== system DvrSimKeybd_cs/Roewe_550_S_Sedan_1/Subsystem/TyreContact To Road Information/Contact To Road Information/AvoidDivisionByZero ==
  In1 : Inport
  Compare To Zero : simulink/Logic and Bit Operations/Compare To Zero  relop===  OutDataTypeStr=uint8
  Constant : Constant  Value=eps
  Product : Product  RndMeth=Zero
  Sum : Sum
  Out1 : Outport
  wires:
  In1/1 -> Compare To Zero/1, Sum/1
  Sum/1 -> Out1/1
  Product/1 -> Sum/2
  Constant/1 -> Product/2
  Compare To Zero/1 -> Product/1

== system DvrSimKeybd_cs/Roewe_550_S_Sedan_1/Subsystem/TyreContact To Road Information/Contact To Road Information/Transformation_PreScan2CarSim ==
  UnitVec_z_CP_CoorSys_PreScan[FL;FR;RL;RR][x;y;z] : Inport
  angles_BODYwrtGLOB_[deg] : Inport  Port=2
  Bus Creator : BusCreator  Inputs=4
  D2R : Gain  Gain=pi/180
  Fcn1 : Fcn  Expr=cos(u(1))*sin(u(2))*sin(u(3))-sin(u(1))*cos(u(3))
  Fcn18 : Fcn  Expr=cos(u(1))*cos(u(2))
  Fcn2 : Fcn  Expr=cos(u(1))*sin(u(2))*cos(u(3))+sin(u(1))*sin(u(3))
  Fcn3 : Fcn  Expr=sin(u(1))*cos(u(2))
  Fcn4 : Fcn  Expr=sin(u(1))*sin(u(2))*sin(u(3))+cos(u(1))*cos(u(3))
  Fcn5 : Fcn  Expr=sin(u(1))*sin(u(2))*cos(u(3))-cos(u(1))*sin(u(3))
  Fcn6 : Fcn  Expr=-sin(u(2))
  Fcn7 : Fcn  Expr=cos(u(2))*sin(u(3))
  Fcn8 : Fcn  Expr=cos(u(2))*cos(u(3))
  Mux2 : Mux  Inputs=9
  Selector : Selector  InputPortWidth=9  IndexOptions=Index vector (dialog)  Indices=[1 2 3]  OutputSizes=1
  Selector1 : Selector  InputPortWidth=9  IndexOptions=Index vector (dialog)  Indices=[4 5 6]  OutputSizes=1
  Selector2 : Selector  InputPortWidth=9  IndexOptions=Index vector (dialog)  Indices=[7 8 9]  OutputSizes=1
  Subsystem : Subsystem
  rot_xyz 2 rot_zyx : Selector  InputPortWidth=3  IndexOptions=Index vector (dialog)  Indices=[3 2 1]  OutputSizes=1
  UnitVec_z_CP_CoorSys _CarSim[FL;FR;RL;RR][x;y;z] : Outport
  wires:
  Fcn18/1 -> Mux2/1
  Fcn3/1 -> Mux2/2
  Fcn6/1 -> Mux2/3
  Fcn1/1 -> Mux2/4
  Fcn4/1 -> Mux2/5
  Fcn7/1 -> Mux2/6
  Fcn2/1 -> Mux2/7
  Fcn5/1 -> Mux2/8
  Fcn8/1 -> Mux2/9
  Mux2/1 -> Selector/1, Selector1/1, Selector2/1  "Inverse RotationMatrix"
  rot_xyz 2 rot_zyx/1 -> Fcn18/1, Fcn3/1, Fcn6/1, Fcn1/1, Fcn4/1, Fcn8/1, Fcn5/1, Fcn2/1, Fcn7/1
  D2R/1 -> rot_xyz 2 rot_zyx/1
  Subsystem/4(UnitVec_z_CP_CoorSys_CarSim[RR][x;y;z]) -> Bus Creator/4
  Subsystem/3(UnitVec_z_CP_CoorSys_CarSim[RL][x;y;z]) -> Bus Creator/3
  Subsystem/2(UnitVec_z_CP_CoorSys_CarSim[FR][x;y;z]) -> Bus Creator/2
  Subsystem/1(UnitVec_z_CP_CoorSys_CarSim[FL][x;y;z]) -> Bus Creator/1
  UnitVec_z_CP_CoorSys_PreScan[FL;FR;RL;RR][x;y;z]/1 -> Subsystem/1(UnitVec_z_CP_CoorSys_PreScan[FL;FR;RL;RR][x;y;z])
  angles_BODYwrtGLOB_[deg]/1 -> D2R/1
  Bus Creator/1 -> UnitVec_z_CP_CoorSys _CarSim[FL;FR;RL;RR][x;y;z]/1
  Selector2/1 -> Subsystem/4(ThirdRow)
  Selector1/1 -> Subsystem/3(SecondRow)
  Selector/1 -> Subsystem/2(FirstRow)

== system DvrSimKeybd_cs/Roewe_550_S_Sedan_1/Subsystem1/CarSim2PreScan_BUS/Steering/AvoidDivisionByZero ==
  In1 : Inport
  Compare To Zero : simulink/Logic and Bit Operations/Compare To Zero  relop===  OutDataTypeStr=uint8
  Constant : Constant  Value=eps
  Product : Product  RndMeth=Zero
  Sum : Sum
  Out1 : Outport
  wires:
  In1/1 -> Compare To Zero/1, Sum/1
  Sum/1 -> Out1/1
  Product/1 -> Sum/2
  Constant/1 -> Product/2
  Compare To Zero/1 -> Product/1

== system DvrSimKeybd_cs/Roewe_550_S_Sedan_1/Subsystem1/CarSim2PreScan_BUS/Wheel/Convert CarSim to PreScan Wheel Position ==
  SprungMass_Pos_Global[x;y;z][m] : Inport
  SprungMass_Angle_Global[x;y;z][deg] : Inport  Port=2
  CarSim_Pos_FL_Wheel[x;y;z][m] : Inport  Port=3
  CarSim_Pos_FR_Wheel[x;y;z][m] : Inport  Port=4
  CarSim_Pos_RL_Wheel[x;y;z][m] : Inport  Port=5
  CarSim_Pos_RR_Wheel[x;y;z][m] : Inport  Port=6
  Bus Creator1 : BusCreator  Inputs=4
  Demux1 : Demux  Outputs=[3 3 3 3]
  Mux1 : Mux
  Transformation_WheelGlobal2WheelLocal : Subsystem
  PreScanWheel_Pos : Outport
  wires:
  SprungMass_Angle_Global[x;y;z][deg]/1 -> Transformation_WheelGlobal2WheelLocal/2(SprungMass_Angle_Global[x;y;z][deg])
  SprungMass_Pos_Global[x;y;z][m]/1 -> Transformation_WheelGlobal2WheelLocal/1(SprungMass_Pos_Global[x;y;z][m])
  CarSim_Pos_RR_Wheel[x;y;z][m]/1 -> Mux1/4
  CarSim_Pos_RL_Wheel[x;y;z][m]/1 -> Mux1/3
  CarSim_Pos_FR_Wheel[x;y;z][m]/1 -> Mux1/2
  CarSim_Pos_FL_Wheel[x;y;z][m]/1 -> Mux1/1
  Mux1/1 -> Transformation_WheelGlobal2WheelLocal/3(Wheels_Pos_Global[x;y;z][m])
  Bus Creator1/1 -> PreScanWheel_Pos/1  "Linear"
  Demux1/4 -> Bus Creator1/4  "Pos_RR_Wheel_CoorSys_V[x;y;z][m]"
  Demux1/3 -> Bus Creator1/3  "Pos_RL_Wheel_CoorSys_V[x;y;z][m]"
  Demux1/2 -> Bus Creator1/2  "Pos_FR_Wheel_CoorSys_V[x;y;z][m]"
  Demux1/1 -> Bus Creator1/1  "Pos_FL_Wheel_CoorSys_V[x;y;z][m]"
  Transformation_WheelGlobal2WheelLocal/1(Pos_[FL;FR;RL;RR]_Wheel_CoorSys_V[x;y;z][m]) -> Demux1/1

== system DvrSimKeybd_cs/Roewe_550_S_Sedan_1/Subsystem1/CarSim2PreScan_BUS/Wheel/Convert CarSim to PreScan Wheel Rotation ==
  CarSim_Angle_FL_Wheel_CoorSys_V[deg;rev;deg] : Inport
  CarSim_Angle_FR_Wheel_CoorSys_V[deg;rev;deg] : Inport  Port=2
  CarSim_Angle_RL_Wheel_CoorSys_V[deg;rev;deg] : Inport  Port=3
  CarSim_Angle_RR_Wheel_CoorSys_V[deg;rev;deg] : Inport  Port=4
  Angle_Vehicle[x;y;z][deg] : Inport  Port=5
  Bus Creator{,1,3..4} (4 alike) : BusCreator  Inputs=3
  Bus Creator2 : BusCreator  Inputs=4
  Demux{,1..4} (5 alike) : Demux  Outputs=3
  Rev2D{,1..3} (4 alike) : Gain  Gain=360
  Sum{1..4} (4 alike) : Sum  Inputs=+-
  Terminator : Terminator
  Terminator1 : Terminator
  PreScanWheel_Rot : Outport
  wires:
  [VehicleRoll_deg] -> Sum3/2
  Sum3/1 -> Bus Creator4/1  "Angle_Camber_RR_Wheel_CoorSys_V[deg]"
  [VehicleRoll_deg] -> Sum2/2
  Sum1/1 -> Bus Creator1/1  "Angle_Camber_FR_Wheel_CoorSys_V[deg]"
  [VehicleRoll_deg] -> Sum1/2
  [VehicleRoll_deg] -> Sum4/2
  Demux4/3 -> Terminator1/1
  Demux4/2 -> Terminator/1
  Demux4/1 -> [VehicleRoll_deg]
  Angle_Vehicle[x;y;z][deg]/1 -> Demux4/1
  Rev2D3/1 -> Bus Creator4/2  "Angle_Rot_RR_Wheel[deg]"
  Rev2D2/1 -> Bus Creator3/2  "Angle_Rot_RL_Wheel[deg]"
  Rev2D1/1 -> Bus Creator1/2  "Angle_Rot_FR_Wheel[deg]"
  Rev2D/1 -> Bus Creator/2  "Angle_Rot_FL_Wheel[deg]"
  CarSim_Angle_RR_Wheel_CoorSys_V[deg;rev;deg]/1 -> Demux3/1
  CarSim_Angle_RL_Wheel_CoorSys_V[deg;rev;deg]/1 -> Demux2/1
  CarSim_Angle_FR_Wheel_CoorSys_V[deg;rev;deg]/1 -> Demux1/1
  Demux/1 -> Sum4/1  "CarSImAngle_Camber_FL_Wheel_CoorSys_V[deg]"
  Bus Creator2/1 -> PreScanWheel_Rot/1  "Angualr"
  Bus Creator4/1 -> Bus Creator2/4  "Rot_RR_Wheel_CoorSys_V[x;y;z][deg]"
  Bus Creator3/1 -> Bus Creator2/3  "Rot_RL_Wheel_CoorSys_V[x;y;z][deg]"
  Bus Creator1/1 -> Bus Creator2/2  "Rot_FR_Wheel_CoorSys_V[x;y;z][deg]"
  Bus Creator/1 -> Bus Creator2/1  "Rot_FL_Wheel_CoorSys_V[x;y;z][deg]"
  Demux3/3 -> Bus Creator4/3  "Angle_Toe_RR_Wheel_CoorSys_V[deg]"
  Demux1/3 -> Bus Creator1/3  "Angle_Toe_FR_Wheel_CoorSys_V[deg]"
  Demux2/3 -> Bus Creator3/3  "Angle_Toe_RL_Wheel_CoorSys_V[deg]"
  Sum2/1 -> Bus Creator3/1  "Angle_Camber_RL_Wheel_CoorSys_V[deg]"
  Sum4/1 -> Bus Creator/1  "Angle_Camber_FL_Wheel_CoorSys_V[deg]"
  Demux3/2 -> Rev2D3/1  "Angle_Rot_RR_Wheel[rev]"
  Demux3/1 -> Sum3/1  "Angle_Camber_RR_Wheel_CoorSys_V[deg]"
  Demux2/2 -> Rev2D2/1  "Angle_Rot_RL_Wheel[rev]"
  Demux2/1 -> Sum2/1  "Angle_Camber_RL_Wheel_CoorSys_V[deg]"
  Demux1/2 -> Rev2D1/1  "Angle_Rot_FR_Wheel[rev]"
  Demux1/1 -> Sum1/1  "Angle_Camber_FR_Wheel_CoorSys_V[deg]"
  Demux/3 -> Bus Creator/3  "Angle_Toe_FL_Wheel_CoorSys_V[deg]"
  Demux/2 -> Rev2D/1  "Angle_Rot_FL_Wheel[rev]"
  CarSim_Angle_FL_Wheel_CoorSys_V[deg;rev;deg]/1 -> Demux/1

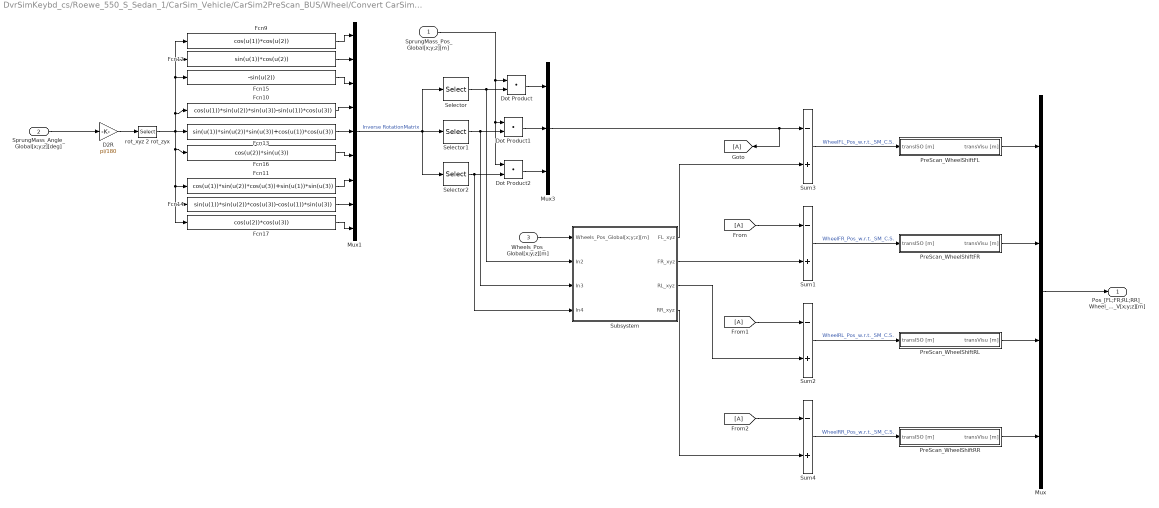
== system DvrSimKeybd_cs/Roewe_550_S_Sedan_1/CarSim_Vehicle/CarSim2PreScan_BUS/Wheel/Convert CarSim to PreScan Wheel Position/Transformation_WheelGlobal2WheelLocal ==
  SprungMass_Pos_Global[x;y;z][m] : Inport
  SprungMass_Angle_Global[x;y;z][deg] : Inport  Port=2
  Wheels_Pos_Global[x;y;z][m] : Inport  Port=3
  D2R : Gain  Gain=pi/180
  Dot Product : DotProduct  InputSameDT=on  OutDataTypeStr=Inherit: Inherit via internal rule
  Dot Product1 : DotProduct  InputSameDT=on  OutDataTypeStr=Inherit: Inherit via internal rule
  Dot Product2 : DotProduct  InputSameDT=on  OutDataTypeStr=Inherit: Inherit via internal rule
  Fcn10 : Fcn  Expr=cos(u(1))*sin(u(2))*sin(u(3))-sin(u(1))*cos(u(3))
  Fcn11 : Fcn  Expr=cos(u(1))*sin(u(2))*cos(u(3))+sin(u(1))*sin(u(3))
  Fcn12 : Fcn  Expr=sin(u(1))*cos(u(2))
  Fcn13 : Fcn  Expr=sin(u(1))*sin(u(2))*sin(u(3))+cos(u(1))*cos(u(3))
  Fcn14 : Fcn  Expr=sin(u(1))*sin(u(2))*cos(u(3))-cos(u(1))*sin(u(3))
  Fcn15 : Fcn  Expr=-sin(u(2))
  Fcn16 : Fcn  Expr=cos(u(2))*sin(u(3))
  Fcn17 : Fcn  Expr=cos(u(2))*cos(u(3))
  Fcn9 : Fcn  Expr=cos(u(1))*cos(u(2))
  Mux : Mux
  Mux1 : Mux  Inputs=9
  Mux3 : Mux  Inputs=3
  PreScan_WheelShiftFL : Subsystem  mask(Translation node configuration){tp=Rear-Left Wheel}
      mask prompts: tp "Type"
      mask init:
      | x_ini_VRML = 2.701790; 
      | y_ini_VRML = 0.665750; 
      | z_ini_VRML = 0.317714;
      mask TypeOptions tp: Front-Left Wheel | Front-Right Wheel | Rear-Left Wheel | Rear-Right Wheel | Left Seat | Right Seat
  PreScan_WheelShiftFR : Subsystem  mask(Translation node configuration){tp=Rear-Right Wheel}
      mask prompts: tp "Type"
      mask init:
      | x_ini_VRML = 2.701790; 
      | y_ini_VRML = -0.665750; 
      | z_ini_VRML = 0.317714;
      mask TypeOptions tp: Front-Left Wheel | Front-Right Wheel | Rear-Left Wheel | Rear-Right Wheel | Left Seat | Right Seat
  PreScan_WheelShiftRL : Subsystem  mask(Translation node configuration){tp=Front-Left Wheel}
      mask prompts: tp "Type"
      mask init:
      | x_ini_VRML = 0.000000; 
      | y_ini_VRML = 0.665750; 
      | z_ini_VRML = 0.317714;
      mask TypeOptions tp: Front-Left Wheel | Front-Right Wheel | Rear-Left Wheel | Rear-Right Wheel | Left Seat | Right Seat
  PreScan_WheelShiftRR : Subsystem  mask(Translation node configuration){tp=Front-Right Wheel}
      mask prompts: tp "Type"
      mask init:
      | x_ini_VRML = 0.000000; 
      | y_ini_VRML = -0.665750; 
      | z_ini_VRML = 0.317714;
      mask TypeOptions tp: Front-Left Wheel | Front-Right Wheel | Rear-Left Wheel | Rear-Right Wheel | Left Seat | Right Seat
  Selector : Selector  InputPortWidth=9  IndexOptions=Index vector (dialog)  Indices=[1 2 3]  OutputSizes=1
  Selector1 : Selector  InputPortWidth=9  IndexOptions=Index vector (dialog)  Indices=[4 5 6]  OutputSizes=1
  Selector2 : Selector  InputPortWidth=9  IndexOptions=Index vector (dialog)  Indices=[7 8 9]  OutputSizes=1
  Subsystem : Subsystem
  Sum{1..4} (4 alike) : Sum  Inputs=-+
  rot_xyz 2 rot_zyx : Selector  InputPortWidth=3  IndexOptions=Index vector (dialog)  Indices=[3 2 1]  OutputSizes=1
  Pos_[FL;FR;RL;RR]_Wheel_CoorSys_V[x;y;z][m] : Outport
  wires:
  PreScan_WheelShiftFL/1(transVisu [m]) -> Mux/1
  PreScan_WheelShiftRL/1(transVisu [m]) -> Mux/3
  PreScan_WheelShiftFR/1(transVisu [m]) -> Mux/2
  D2R/1 -> rot_xyz 2 rot_zyx/1
  Mux/1 -> Pos_[FL;FR;RL;RR]_Wheel_CoorSys_V[x;y;z][m]/1
  PreScan_WheelShiftRR/1(transVisu [m]) -> Mux/4
  [A] -> Sum4/1
  [A] -> Sum2/1
  [A] -> Sum1/1
  Sum4/1 -> PreScan_WheelShiftRR/1(transISO [m])  "WheelRR_Pos_w.r.t._SM_C.S."
  Sum2/1 -> PreScan_WheelShiftRL/1(transISO [m])  "WheelRL_Pos_w.r.t._SM_C.S."
  Sum1/1 -> PreScan_WheelShiftFR/1(transISO [m])  "WheelFR_Pos_w.r.t._SM_C.S."
  Subsystem/4(RR_xyz) -> Sum4/2
  Subsystem/3(RL_xyz) -> Sum2/2
  Subsystem/2(FR_xyz) -> Sum1/2
  Subsystem/1(FL_xyz) -> Sum3/2
  Wheels_Pos_Global[x;y;z][m]/1 -> Subsystem/1(Wheels_Pos_Global[x;y;z][m])
  Sum3/1 -> PreScan_WheelShiftFL/1(transISO [m])  "WheelFL_Pos_w.r.t._SM_C.S."
  SprungMass_Angle_Global[x;y;z][deg]/1 -> D2R/1
  Mux3/1 -> [A], Sum3/1
  rot_xyz 2 rot_zyx/1 -> Fcn16/1, Fcn11/1, Fcn14/1, Fcn17/1, Fcn13/1, Fcn10/1, Fcn15/1, Fcn12/1, Fcn9/1
  Dot Product1/1 -> Mux3/2
  Dot Product2/1 -> Mux3/3
  Selector2/1 -> Subsystem/4(In4), Dot Product2/2
  Selector1/1 -> Subsystem/3(In3), Dot Product1/2
  Dot Product/1 -> Mux3/1
  SprungMass_Pos_Global[x;y;z][m]/1 -> Dot Product/1, Dot Product2/1, Dot Product1/1
  Selector/1 -> Subsystem/2(In2), Dot Product/2
  Mux1/1 -> Selector2/1, Selector1/1, Selector/1  "Inverse RotationMatrix"
  Fcn17/1 -> Mux1/9
  Fcn14/1 -> Mux1/8
  Fcn11/1 -> Mux1/7
  Fcn16/1 -> Mux1/6
  Fcn13/1 -> Mux1/5
  Fcn10/1 -> Mux1/4
  Fcn15/1 -> Mux1/3
  Fcn12/1 -> Mux1/2
  Fcn9/1 -> Mux1/1

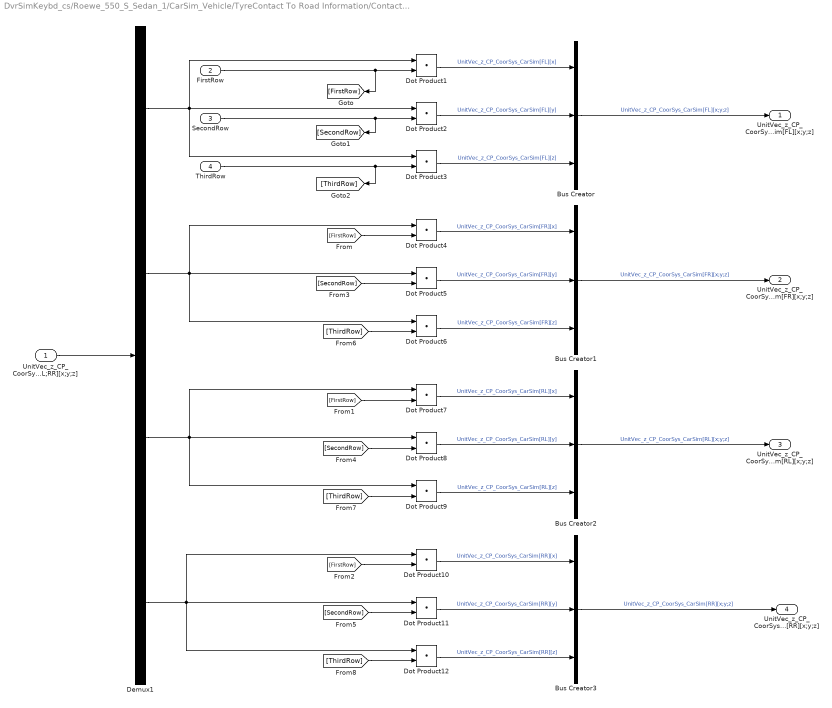
== system DvrSimKeybd_cs/Roewe_550_S_Sedan_1/CarSim_Vehicle/TyreContact To Road Information/Contact To Road Information/Transformation_PreScan2CarSim/Subsystem ==
  UnitVec_z_CP_CoorSys_PreScan[FL;FR;RL;RR][x;y;z] : Inport
  FirstRow : Inport  Port=2
  SecondRow : Inport  Port=3
  ThirdRow : Inport  Port=4
  Bus Creator{,1..3} (4 alike) : BusCreator  Inputs=3
  Demux1 : Demux  Outputs=[3 3 3 3]
  Dot Product{1..12} (12 alike) : DotProduct  InputSameDT=on  OutDataTypeStr=Inherit: Inherit via internal rule
  UnitVec_z_CP_CoorSys_CarSim[FL][x;y;z] : Outport
  UnitVec_z_CP_CoorSys_CarSim[FR][x;y;z] : Outport  Port=2
  UnitVec_z_CP_CoorSys_CarSim[RL][x;y;z] : Outport  Port=3
  UnitVec_z_CP_CoorSys_CarSim[RR][x;y;z] : Outport  Port=4
  wires:
  [ThirdRow] -> Dot Product12/2
  [ThirdRow] -> Dot Product9/2
  [ThirdRow] -> Dot Product6/2
  [SecondRow] -> Dot Product11/2
  [SecondRow] -> Dot Product8/2
  [SecondRow] -> Dot Product5/2
  FirstRow/1 -> [FirstRow], Dot Product1/2
  [FirstRow] -> Dot Product10/2
  [FirstRow] -> Dot Product7/2
  [FirstRow] -> Dot Product4/2
  Demux1/4 -> Dot Product12/1, Dot Product10/1, Dot Product11/1
  Demux1/3 -> Dot Product9/1, Dot Product7/1, Dot Product8/1
  Demux1/2 -> Dot Product6/1, Dot Product5/1, Dot Product4/1
  Demux1/1 -> Dot Product3/1, Dot Product2/1, Dot Product1/1
  Bus Creator3/1 -> UnitVec_z_CP_CoorSys_CarSim[RR][x;y;z]/1  "UnitVec_z_CP_CoorSys_CarSim[RR][x;y;z]"
  Dot Product11/1 -> Bus Creator3/2  "UnitVec_z_CP_CoorSys_CarSim[RR][y]"
  Dot Product12/1 -> Bus Creator3/3  "UnitVec_z_CP_CoorSys_CarSim[RR][z]"
  Dot Product10/1 -> Bus Creator3/1  "UnitVec_z_CP_CoorSys_CarSim[RR][x]"
  Bus Creator2/1 -> UnitVec_z_CP_CoorSys_CarSim[RL][x;y;z]/1  "UnitVec_z_CP_CoorSys_CarSim[RL][x;y;z]"
  Dot Product8/1 -> Bus Creator2/2  "UnitVec_z_CP_CoorSys_CarSim[RL][y]"
  Dot Product9/1 -> Bus Creator2/3  "UnitVec_z_CP_CoorSys_CarSim[RL][z]"
  Dot Product7/1 -> Bus Creator2/1  "UnitVec_z_CP_CoorSys_CarSim[RL][x]"
  Bus Creator1/1 -> UnitVec_z_CP_CoorSys_CarSim[FR][x;y;z]/1  "UnitVec_z_CP_CoorSys_CarSim[FR][x;y;z]"
  Dot Product5/1 -> Bus Creator1/2  "UnitVec_z_CP_CoorSys_CarSim[FR][y]"
  Dot Product6/1 -> Bus Creator1/3  "UnitVec_z_CP_CoorSys_CarSim[FR][z]"
  Dot Product4/1 -> Bus Creator1/1  "UnitVec_z_CP_CoorSys_CarSim[FR][x]"
  Bus Creator/1 -> UnitVec_z_CP_CoorSys_CarSim[FL][x;y;z]/1  "UnitVec_z_CP_CoorSys_CarSim[FL][x;y;z]"
  Dot Product2/1 -> Bus Creator/2  "UnitVec_z_CP_CoorSys_CarSim[FL][y]"
  Dot Product3/1 -> Bus Creator/3  "UnitVec_z_CP_CoorSys_CarSim[FL][z]"
  Dot Product1/1 -> Bus Creator/1  "UnitVec_z_CP_CoorSys_CarSim[FL][x]"
  UnitVec_z_CP_CoorSys_PreScan[FL;FR;RL;RR][x;y;z]/1 -> Demux1/1
  ThirdRow/1 -> [ThirdRow], Dot Product3/2
  SecondRow/1 -> [SecondRow], Dot Product2/2
